simulink model "wiper_old"  (R2022b)
settings: Solver=FixedStepDiscrete  StartTime=0.0  StopTime=10.0  FixedStep=0.1  RelTol=1e-3
libraries: simulink x1
settings Model: Creator=Yalaguresh  LastModifiedBy=Yalaguresh
settings OptimizationCC: ReuseModelBlockBuffer=on

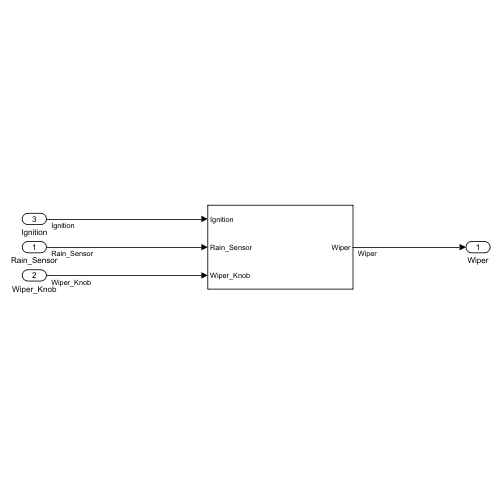
[thumbnail: Simulink's stored preview of the top-level diagram]
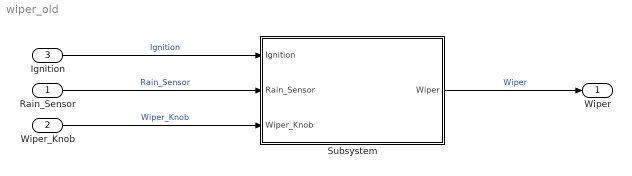
== system wiper_old ==
  Rain_Sensor : Inport
  Wiper_Knob : Inport  Port=2
  Ignition : Inport  Port=3
  Subsystem : Subsystem
  Wiper : Outport
  wires:
  Ignition/1 -> Subsystem/1(Ignition)  "Ignition"
  Rain_Sensor/1 -> Subsystem/2(Rain_Sensor)  "Rain_Sensor"
  Wiper_Knob/1 -> Subsystem/3(Wiper_Knob)  "Wiper_Knob"
  Subsystem/1(Wiper) -> Wiper/1  "Wiper"

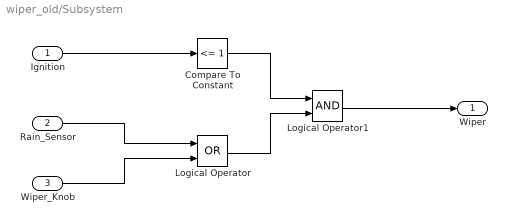
== system wiper_old/Subsystem ==
  Ignition : Inport
  Rain_Sensor : Inport  Port=2
  Wiper_Knob : Inport  Port=3
  Compare To Constant : simulink/Logic and Bit Operations/Compare To Constant  relop=<=  const=1  OutDataTypeStr=boolean
  Logical Operator : Logic  Operator=OR  AllPortsSameDT=off  OutDataTypeStr=boolean
  Logical Operator1 : Logic  AllPortsSameDT=off  OutDataTypeStr=boolean
  Wiper : Outport
  wires:
  Compare To Constant/1 -> Logical Operator1/1
  Logical Operator/1 -> Logical Operator1/2
  Ignition/1 -> Compare To Constant/1
  Logical Operator1/1 -> Wiper/1
  Rain_Sensor/1 -> Logical Operator/1
  Wiper_Knob/1 -> Logical Operator/2
